simulink model "mavsim_chap10_model"  (R2015b)
settings: Solver=ode45  StartTime=0.0  StopTime=400  RelTol=1e-3
InitFcn:
  | param_chap10
undefined symbols (not defined in the file or in its folder): drawPathError, P, path_follow, path_manager_chap10
settings Model: Creator=beard  LastModifiedBy=magiccjae
settings DataIOCC: SaveFormat=Array  SignalLoggingSaveFormat=ModelDataLogs
settings OptimizationCC: ExpressionDepthLimit=2147483647  InitFltsAndDblsToZero=on
settings DebuggingCC: UnderspecifiedInitializationDetection=Classic  MergeDetectMultiDrivingBlocksExec=none  SolverPrmCheckMsg=warning  FcnCallInpInsideContextMsg=UseLocalSettings  StateNameClashWarn=warning
settings HardwareCC: ProdBitPerPointer=32  ProdLargestAtomicFloat=None  ProdIntDivRoundTo=Undefined  ProdEndianess=Unspecified  ProdWordSize=32  ProdHWDeviceType=32-bit Generic
settings SFSimCC: SimParseCustomCode=off
settings GRTTargetCC: GeneratePreprocessorConditionals=Disable all  CombineOutputUpdateFcns=off  GRTInterface=on
settings ConfigComp: CovModelRefEnable=Off  CovSFcnEnable=off

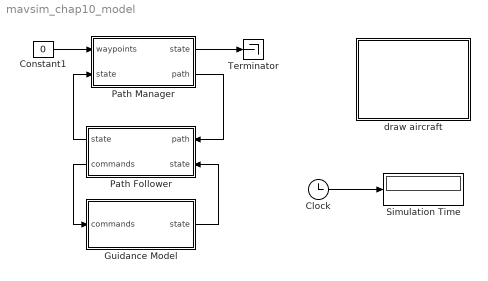
== system mavsim_chap10_model ==
  Clock : Clock
  Constant1 : Constant  Value=0
  Guidance Model : Subsystem
  Path Follower : Subsystem
  Path Manager : Subsystem
  Simulation Time : Display
  Terminator : Terminator
  draw aircraft : Subsystem
      mask Display: image(imread('predator.jpg'))
  wires:
  Clock/1 -> Simulation Time/1
  Path Manager/2(path) -> Path Follower/1(path)
  Path Follower/2(commands) -> Guidance Model/1(commands)
  Guidance Model/1(state) -> Path Follower/2(state)
  Constant1/1 -> Path Manager/1(waypoints)
  Path Follower/1("state ") -> Path Manager/2(state)
  Path Manager/1("state ") -> Terminator/1

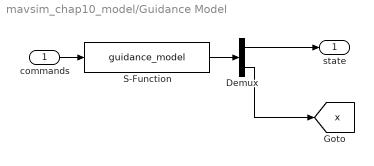
== system mavsim_chap10_model/Guidance Model ==
  commands : Inport
  Demux : Demux  Outputs=[16;12]
  S-Function : S-Function  FunctionName=guidance_model  Parameters=P  SFunctionDeploymentMode=off  EnableBusSupport=off
  state : Outport
  tag scope: x=global
  wires:
  commands/1 -> S-Function/1
  S-Function/1 -> Demux/1
  Demux/1 -> state/1
  Demux/2 -> [x]

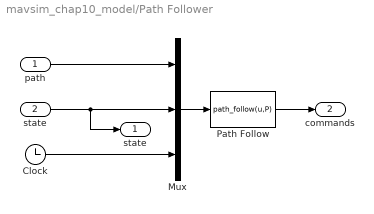
== system mavsim_chap10_model/Path Follower ==
  path : Inport
  state : Inport  Port=2
  Clock : Clock
  Mux : Mux  Inputs=3
  Path Follow : MATLABFcn  MATLABFcn=path_follow(u,P)  OutputDimensions=4  SampleTime=P.Ts
  "state " : Outport
  commands : Outport  Port=2
  wires:
  Path Follow/1 -> commands/1
  Mux/1 -> Path Follow/1
  path/1 -> Mux/1
  Clock/1 -> Mux/3
  state/1 -> Mux/2, "state "/1

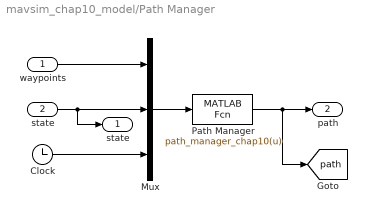
== system mavsim_chap10_model/Path Manager ==
  waypoints : Inport
  state : Inport  Port=2
  Clock : Clock
  Mux : Mux  Inputs=3
  Path Manager : MATLABFcn  MATLABFcn=path_manager_chap10(u)  OutputDimensions=13  SampleTime=P.Ts
  "state " : Outport
  path : Outport  Port=2
  tag scope: path=global
  wires:
  Path Manager/1 -> path/1, [path]
  Mux/1 -> Path Manager/1
  Clock/1 -> Mux/3
  state/1 -> Mux/2, "state "/1
  waypoints/1 -> Mux/1

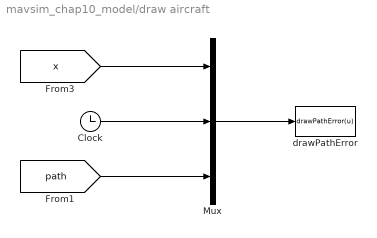
== system mavsim_chap10_model/draw aircraft ==
  Clock : Clock
  Mux : Mux  Inputs=3
  drawPathError : MATLABFcn  MATLABFcn=drawPathError(u)  OutputDimensions=0  SampleTime=0.1
  wires:
  Clock/1 -> Mux/2
  [x] -> Mux/1
  Mux/1 -> drawPathError/1
  [path] -> Mux/3
